simulink library "pm_mfi"  (R2021a)
settings: Solver=VariableStepAuto  StartTime=0.0  StopTime=10.0  RelTol=1e-3
settings Model: Creator=errorput  LastModifiedBy=errorput

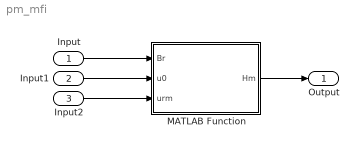
== system pm_mfi ==
  Input : Inport
  Input1 : Inport  Port=2
  Input2 : Inport  Port=3
  MATLAB Function : MATLAB Function  TreatAsAtomicUnit=on
  Output : Outport
  wires:
  Input/1 -> MATLAB Function/1(Br)
  Input2/1 -> MATLAB Function/3(urm)
  Input1/1 -> MATLAB Function/2(u0)
  MATLAB Function/1(Hm) -> Output/1

== matlab function pm_mfi/MATLAB Function ==
  data: Br input; Hm output; u0 input; urm input
function Hm  = pm_mfi(Br,u0,urm)
%UNTITLED2 计算永磁体主极磁场强度
%   Br     剩余磁通密度
%   u0     空气磁导率
%   urm    相对磁导率
Hm = Br/ 2 * u0 * urm;
end
